simulink model "Lab2"  (Simulink 9.1)
settings: Solver=ode45  StartTime=0.0  StopTime=10  RelTol=1e-3  EnableMultiTasking=on
settings Model: SuppressorTable=22 serialization::archive 11 0 6 0 0 0 1 0  Creator=Aramis  LastModifiedBy=wivill
settings DataIOCC: LimitDataPoints=on  SignalLoggingSaveFormat=ModelDataLogs
settings OptimizationCC: ExpressionDepthLimit=2147483647
settings DebuggingCC: SolverPrmCheckMsg=warning  FcnCallInpInsideContextMsg=warning  StateNameClashWarn=warning

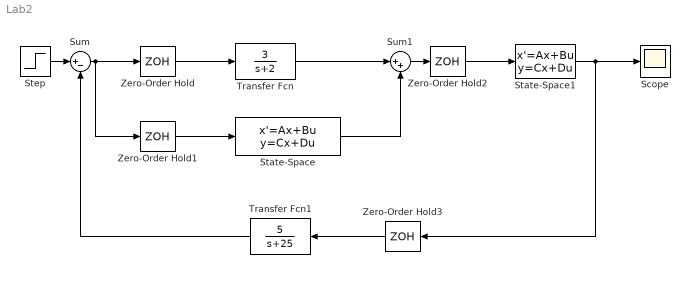
== system Lab2 ==
  Scope : Scope
  State-Space : StateSpace  A=[1 -1;-3 5]  B=[-3;-4]  C=[1 -2]  D=0  InitialCondition=0
  State-Space1 : StateSpace  A=[1 -4 5; -1 7 -1;1 3 4]  B=[1;2;1]  C=[1 -1 1]  D=0  InitialCondition=0
  Step : Step  Time=0  After=0.25  SampleTime=0
  Sum : Sum  Inputs=|+-
  Sum1 : Sum  Inputs=|++
  Transfer Fcn : TransferFcn  Numerator=[3]  Denominator=[1 2]
  Transfer Fcn1 : TransferFcn  Numerator=[5]  Denominator=[1 25]
  Zero-Order Hold{,1..3} (4 alike) : ZeroOrderHold  SampleTime=0.01
  wires:
  Zero-Order Hold/1 -> Transfer Fcn/1
  Sum/1 -> Zero-Order Hold/1, Zero-Order Hold1/1
  Zero-Order Hold1/1 -> State-Space/1
  Transfer Fcn/1 -> Sum1/1
  State-Space/1 -> Sum1/2
  Sum1/1 -> Zero-Order Hold2/1
  Zero-Order Hold2/1 -> State-Space1/1
  State-Space1/1 -> Zero-Order Hold3/1, Scope/1
  Zero-Order Hold3/1 -> Transfer Fcn1/1
  Transfer Fcn1/1 -> Sum/2
  Step/1 -> Sum/1
